simulink model "Middle_Ear_Filter_fil"  (R2019b)
settings: Solver=VariableStepAuto  StartTime=0.0  StopTime=testtime  RelTol=1e-3
InitFcn:
  | Middle_Ear_Test_Parameters
StopFcn:
  | Verify_Middle_Ear_fil
undefined symbols (not defined in the file or in its folder): dfilt, Fs, megainmax, MEscale
libraries: dsparch4 x2, dspsrcs4 x2, simulink x1, fillib x1
settings Model: Creator=mblun  LastModifiedBy=t96f346
settings OptimizationCC: BlockReduction=off  ConditionallyExecuteInputs=off  DefaultParameterBehavior=Inlined
settings DebuggingCC: AlgebraicLoopMsg=error
settings HardwareCC: ProdBitPerPointer=32  ProdBitPerSizeT=32  ProdBitPerPtrDiffT=32  ProdLargestAtomicFloat=None  ProdIntDivRoundTo=Undefined  ProdEndianess=Unspecified  ProdWordSize=32  ProdHWDeviceType=ASIC/FPGA->ASIC/FPGA  TargetBitPerPointer=64  TargetBitPerSizeT=64  TargetBitPerPtrDiffT=64  TargetLongLongMode=on  TargetIntDivRoundTo=Zero  TargetEndianess=LittleEndian  TargetWordSize=64  TargetHWDeviceType=Custom Processor->MATLAB Host Computer  ProdEqTarget=off
settings SFSimCC: CustomCodeUndefinedFunction=UseInterfaceOnly

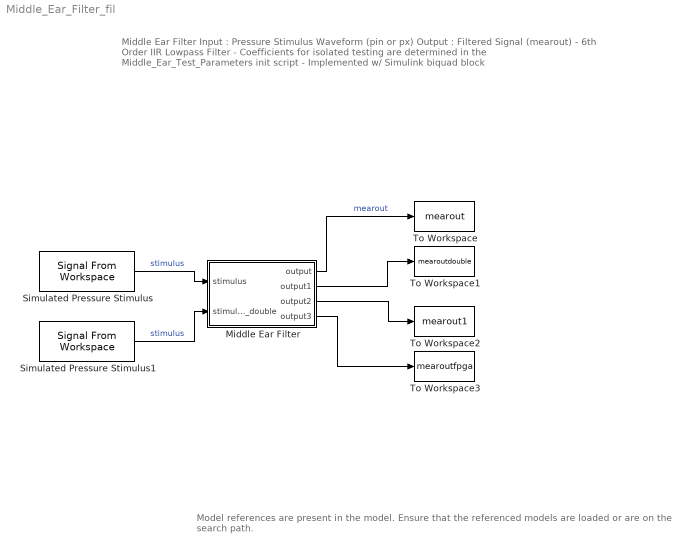
== system Middle_Ear_Filter_fil ==
  note: Middle Ear Filter
      |
      | Input : Pressure Stimulus Waveform (pin or px)
      |
      | Output : Filtered Signal (mearout)
      |
      | - 6th Order IIR Lowpass Filter
      |
      | - Coefficients for isolated testing are determined in the Middle_Ear_Test_Parameters init script
      |
      | - Implemented w/ Simulink biquad block
  note: Model references are present in the model. Ensure that the referenced models are loaded or are on the search path.
  Middle Ear Filter : Subsystem
  Simulated Pressure Stimulus : dspsrcs4/Signal From Workspace  X=RxSignal  Ts=1/Fs  nsamps=1  OutputAfterFinalValue=Setting to zero  ignoreOrWarnInputAndFrameLengths=off  OutputFrames=off
  Simulated Pressure Stimulus1 : dspsrcs4/Signal From Workspace  X=RxSignalDouble  Ts=1/Fs  nsamps=1  OutputAfterFinalValue=Setting to zero  ignoreOrWarnInputAndFrameLengths=off  OutputFrames=off
  To Workspace : ToWorkspace  VariableName=mearout  SampleTime=-1
      settings: Save2DSignal=2-D array (concatenate along first dimension)
  To Workspace1 : ToWorkspace  VariableName=mearoutdouble  SampleTime=-1
      settings: Save2DSignal=2-D array (concatenate along first dimension)
  To Workspace2 : ToWorkspace  VariableName=mearout1  SampleTime=-1
      settings: Save2DSignal=2-D array (concatenate along first dimension)
  To Workspace3 : ToWorkspace  VariableName=mearoutfpga  SampleTime=-1
      settings: Save2DSignal=2-D array (concatenate along first dimension)
  wires:
  Middle Ear Filter/3(output2) -> To Workspace2/1
  Middle Ear Filter/2(output1) -> To Workspace1/1
  Simulated Pressure Stimulus1/1 -> Middle Ear Filter/2(stimulus_double)  "stimulus"
  Middle Ear Filter/1(output) -> To Workspace/1  "mearout"
  Simulated Pressure Stimulus/1 -> Middle Ear Filter/1(stimulus)  "stimulus"
  Middle Ear Filter/4(output3) -> To Workspace3/1

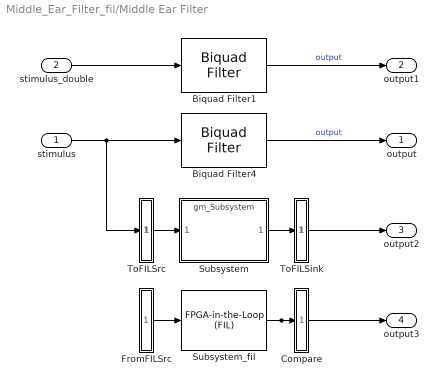
== system Middle_Ear_Filter_fil/Middle Ear Filter ==
  stimulus : Inport
  stimulus_double : Inport  Port=2
  Biquad Filter1 : dsparch4/Biquad Filter  FilterSource=Dialog parameters  CoeffSource=Specify via dialog  FilterObject=dfilt.df2tsos([1 0.3 0.4],[1 0.1 0.2])  IIRFiltStruct=Direct form I  BiQuadCoeffs=MEcoeffs  ScaleValues=[1 1 1 1/megainmax]  IC=0  ICnum=0  ICden=0  a0Flag=Warning  optimizeScaleValues=on  ScaleValueMode=Specify via input port (g)  roundingMode=Floor  overflowMode=on  scaleValueFracLength=14  denProdOutputFracLength=30  denAccumFracLength=30  secondMemoryFracLength=15
      settings: SourceProductName=DSP System Toolbox
  Biquad Filter4 : dsparch4/Biquad Filter  FilterSource=Dialog parameters  CoeffSource=Specify via dialog  FilterObject=dfilt.df2tsos([1 0.3 0.4],[1 0.1 0.2])  IIRFiltStruct=Direct form I  BiQuadCoeffs=MEcoeffs  ScaleValues=[1 1 1 MEscale]  IC=0  ICnum=0  ICden=0  a0Flag=Warning  optimizeScaleValues=on  ScaleValueMode=Specify via input port (g)  roundingMode=Floor  overflowMode=on  scaleValueFracLength=14  denProdOutputFracLength=30  denAccumFracLength=30  secondMemoryFracLength=15
      settings: SourceProductName=DSP System Toolbox
  Compare : Subsystem
      mask Display: disp('')
  FromFILSrc : Subsystem
      mask Display: disp('')
  Subsystem : ModelReference  ModelNameDialog=gm_Subsystem  SimulationMode=Normal  VariantControl=HDLC_internal_variant_GeneratedDUT  ModelReferenceVersion=1.19
  Subsystem_fil : fillib/FPGA-in-the-Loop (FIL)  ForceInterfaceUpdate=0.91338
      settings: SourceProductName=HDL Coder  SourceProductBaseCode=HD
  ToFILSink : Subsystem
      mask Display: disp('')
  ToFILSrc : Subsystem
      mask Display: disp('')
  output : Outport  VectorParamsAs1DForOutWhenUnconnected=off
  output1 : Outport  Port=2  VectorParamsAs1DForOutWhenUnconnected=off
  output2 : Outport  Port=3  VectorParamsAs1DForOutWhenUnconnected=off
  output3 : Outport  Port=4  VectorParamsAs1DForOutWhenUnconnected=off
  wires:
  stimulus_double/1 -> Biquad Filter1/1
  Biquad Filter1/1 -> output1/1  "output"
  Biquad Filter4/1 -> output/1  "output"
  stimulus/1 -> Biquad Filter4/1, ToFILSrc/1(in1)
  ToFILSrc/1(out1) -> Subsystem/1
  Subsystem/1 -> ToFILSink/1(in1)
  ToFILSink/1(out1) -> output2/1
  FromFILSrc/1(out1) -> Subsystem_fil/1
  Subsystem_fil/1 -> output3/1, Compare/1(in1)

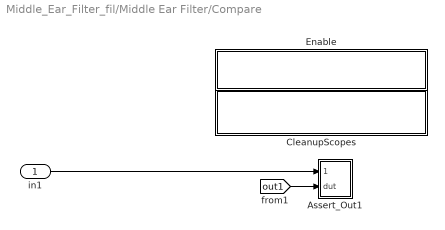
== system Middle_Ear_Filter_fil/Middle Ear Filter/Compare ==
  in1 : Inport
  Assert_Out1 : Subsystem  mask{ToleranceValue=1e-07}
  CleanupScopes : Subsystem
      settings: OpenFcn=|
      | blkName = gcb; %self block
      | idx = regexp(blkName, '/CleanupScopes$', 'once');
      | blkParent = blkName(1:idx-1);
      | blks=find_system(blkParent, 'LookUnderMasks', 'all','blocktype', 'Scope');
      | for itr = 1:length(blks)
      | 	 hScopeCfg = get_param(blks{itr},'ScopeConfiguration');
      | 	 hScopeCfg.Visible = ~ hScopeCfg.Visible;
      | end
      | drawnow;
      mask Display: fprintf(message('hdlcoder:cosim:vnl_dblclick').getString());
  Enable : Subsystem
      settings: OpenFcn=|
      | blkName = gcb;
      | idx = regexp(blkName, '/Enable$', 'once');
      | blkParent = blkName(1:idx-1);
      | blks=find_system(blkParent, 'LookUnderMasks', 'all','blocktype', 'Assertion');
      | e = get_param(blks{1}, 'Enabled');
      | if strcmp(e, 'on'), f= 'off';, else, f = 'on';, end
      | for ii=1:length(blks), set_param(blks{ii}, 'Enabled', f);, end
      | set_param(gcb, 'MaskDisplay',['fprintf(message(''hdlcoder:cosim:vnl_dblclick_assertions'',','''',upper(e),'''',').getString())']);
      mask Display: fprintf(message('hdlcoder:cosim:vnl_dblclick_assertions','OFF').getString());
  wires:
  in1/1 -> Assert_Out1/1(cosim)
  [out1] -> Assert_Out1/2(dut)

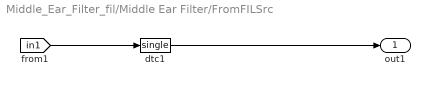
== system Middle_Ear_Filter_fil/Middle Ear Filter/FromFILSrc ==
  dtc1 : DataTypeConversion  OutDataTypeStr=single  SaturateOnIntegerOverflow=on  RndMeth=Zero
  out1 : Outport
  wires:
  [in1] -> dtc1/1
  dtc1/1 -> out1/1

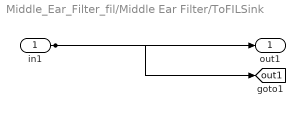
== system Middle_Ear_Filter_fil/Middle Ear Filter/ToFILSink ==
  in1 : Inport
  out1 : Outport
  tag scope: out1=global
  wires:
  in1/1 -> out1/1, [out1]

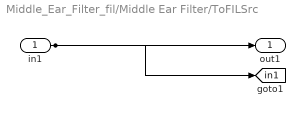
== system Middle_Ear_Filter_fil/Middle Ear Filter/ToFILSrc ==
  in1 : Inport
  out1 : Outport
  tag scope: in1=global
  wires:
  in1/1 -> out1/1, [in1]

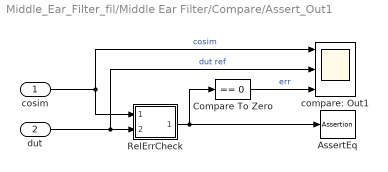
== system Middle_Ear_Filter_fil/Middle Ear Filter/Compare/Assert_Out1 ==
  cosim : Inport
  dut : Inport  Port=2
  AssertEq : Assertion  StopWhenAssertionFail=off
  Compare To Zero : simulink/Logic and Bit Operations/Compare To Zero  relop===  OutDataTypeStr=boolean
  RelErrCheck : Subsystem
  compare: Out1 : Scope  NumInputPorts=3
  wires:
  dut/1 -> compare: Out1/2, RelErrCheck/2(In2)  "dut ref"
  cosim/1 -> compare: Out1/1, RelErrCheck/1(In1)  "cosim"
  RelErrCheck/1(Out1) -> AssertEq/1, Compare To Zero/1
  Compare To Zero/1 -> compare: Out1/3  "err"

== system Middle_Ear_Filter_fil/Middle Ear Filter/Compare/CleanupScopes ==

== system Middle_Ear_Filter_fil/Middle Ear Filter/Compare/Enable ==

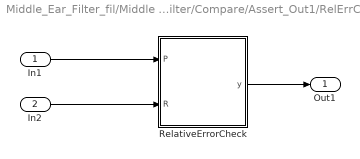
== system Middle_Ear_Filter_fil/Middle Ear Filter/Compare/Assert_Out1/RelErrCheck ==
  In1 : Inport
  In2 : Inport  Port=2
  "RelativeErrorCheck " : MATLAB Function  TreatAsAtomicUnit=on
  Out1 : Outport  VectorParamsAs1DForOutWhenUnconnected=off
  wires:
  In2/1 -> "RelativeErrorCheck "/2(R)
  In1/1 -> "RelativeErrorCheck "/1(P)
  "RelativeErrorCheck "/1(y) -> Out1/1

== matlab function Middle_Ear_Filter_fil/Middle Ear Filter/Compare/Assert_Out1/RelErrCheck/RelativeErrorCheck  ==
  data: P input; y output; R input; ToleranceValue parameter double
% Check if the relative error of R with respect to P is below
% ToleranceValue
% P, R are floating-point
function y = relErrCheck(P,R, ToleranceValue)
    tol = ToleranceValue;
    sz = numel(P);
    assert(sz == numel(R), 'Inputs P and R have different sizes.');
    y = false(1, sz);

    for ii=1:sz
        if (isnan(P(ii)) || isnan(R(ii)))
            if (isnan(P(ii)) && isnan(R(ii)))
                y(ii) = true;
            end
        elseif (isinf(P(ii)) || isinf(R(ii)))
            y(ii) = (P(ii) == R(ii));
        elseif (P(ii) == 0)
            y(ii) = (R(ii) == 0);
        else
            absdiff = abs(P(ii) - R(ii));
            relerr = absdiff/abs(P(ii));
            y(ii) = (relerr <= tol);
        end
    end
end
